simulink model "p1p2p3_Traking_Control"  (R2020b)
settings: Solver=FixedStepDiscrete  StartTime=0.0  StopTime=Inf  FixedStep=0.005  RelTol=1e-3  EnableMultiTasking=on
undefined symbols (not defined in the file or in its folder): DiscIntNeverNeededParam, Send_GUIdata, Writer
libraries: simulink x12, c280xlib x4, c2833xlib x4, dspsrcs4 x2, c2000lib x1
settings Model: ExtModeTrigDuration=8  Creator=Administrator  LastModifiedBy=Administrator
settings DataIOCC: ReturnWorkspaceOutputs=off
settings OptimizationCC: DefaultUnderspecifiedDataType=single  EnhancedBackFolding=on  PassReuseOutputArgsAs=Individual arguments  MaxStackSize=512  OptimizeBlockOrder=speed  DifferentSizesBufferReuse=on  OptimizationCustomize=off  EfficientTunableParamExpr=on
settings DebuggingCC: MultiTaskDSMMsg=none  ParameterTunabilityLossMsg=error  ArithmeticOperatorsInVariantConditions=warning
settings HardwareCC: ProdBitPerChar=16  ProdBitPerInt=16  ProdBitPerPointer=32  ProdBitPerSizeT=32  ProdBitPerPtrDiffT=32  ProdLargestAtomicInteger=Integer  ProdLargestAtomicFloat=None  ProdWordSize=16  ProdLongLongMode=on  ProdHWDeviceType=Texas Instruments->C2000
settings SFSimCC: MATLABDynamicMemAlloc=off  CustomCodeUndefinedFunction=UseInterfaceOnly
settings RTWCC: Description=Embedded Coder  SystemTargetFile=ert.tlc  HardwareBoard=TI Delfino F2833x  TemplateMakefile=ert_default_tmf  GenerateReport=on  Toolchain=Texas Instruments Code Composer Studio (C2000)  IncludeHyperlinkInReport=on  LaunchReport=on  GenerateTraceInfo=on  GenerateTraceReport=on  GenerateTraceReportSl=on  GenerateTraceReportSf=on  GenerateTraceReportEml=on
settings CodeAppCC: ForceParamTrailComments=on  IgnoreCustomStorageClasses=off  OperatorAnnotations=on  SimulinkDataObjDesc=on  SFDataObjDesc=on  InsertBlockDesc=on
settings ERTTargetCC: CodeReplacementLibrary=TI C28x

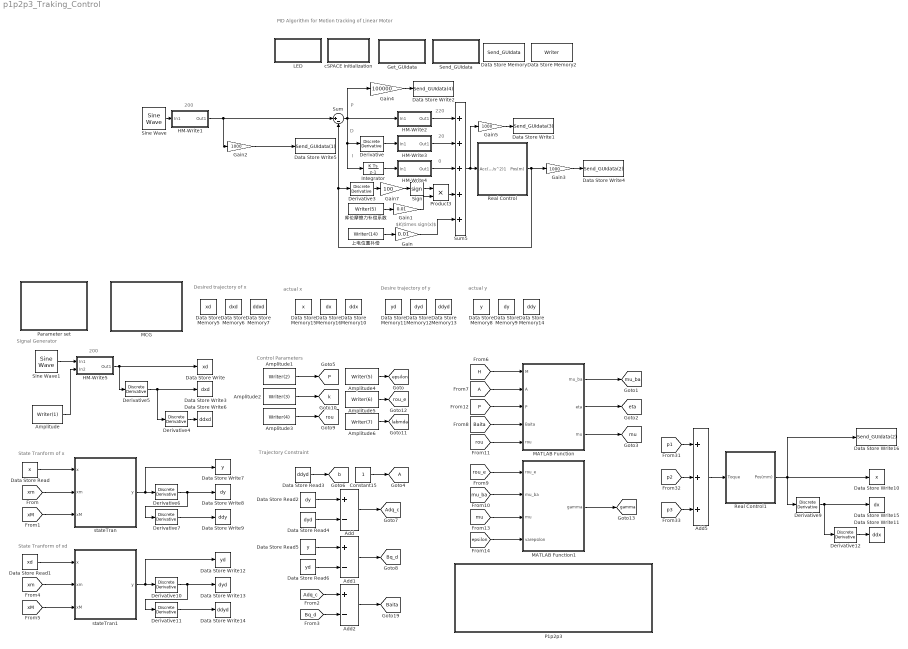
== system p1p2p3_Traking_Control ==
  note: 20
  note: 220
  note: PID Algorithm for Motion tracking of Linear Motor
  note: D
  note: I
  note: 200
  note: P
  note: $K\times sign(x)$
  note: 0
  note: Signal Generator
  note: State Tranform of x
  note: State Tranform of xd
  note: Desired trajectory of x
  note: actual y
  note: Control Parameters
  note: Desire trajectory of y
  note: Trajectory Constraint
  note: actual x
  note: 200
  Add : Sum  Inputs=+-
  Add1 : Sum  Inputs=+-
  Add2 : Sum  Inputs=+-
  Add5 : Sum  Inputs=+++
  Amplitude : DataStoreRead  DataStoreName=Writer  DataStoreElements=Writer(1)
  Amplitude1 : DataStoreRead  DataStoreName=Writer  DataStoreElements=Writer(2)
  Amplitude2 : DataStoreRead  DataStoreName=Writer  DataStoreElements=Writer(3)
  Amplitude3 : DataStoreRead  DataStoreName=Writer  DataStoreElements=Writer(4)
  Amplitude4 : DataStoreRead  DataStoreName=Writer  DataStoreElements=Writer(5)
  Amplitude5 : DataStoreRead  DataStoreName=Writer  DataStoreElements=Writer(6)
  Amplitude6 : DataStoreRead  DataStoreName=Writer  DataStoreElements=Writer(7)
  Constant15 : Constant
  Data Store Memory : DataStoreMemory  DataStoreName=Send_GUIdata  ReadBeforeWriteMsg=warning  WriteAfterWriteMsg=warning  WriteAfterReadMsg=warning  InitialValue=zeros(1,10)  ShowAdditionalParam=off
  Data Store Memory10 : DataStoreMemory  DataStoreName=ddx  ReadBeforeWriteMsg=warning  WriteAfterWriteMsg=warning  WriteAfterReadMsg=warning  ShowAdditionalParam=off
  Data Store Memory11 : DataStoreMemory  DataStoreName=yd  ReadBeforeWriteMsg=warning  WriteAfterWriteMsg=warning  WriteAfterReadMsg=warning  ShowAdditionalParam=off
  Data Store Memory12 : DataStoreMemory  DataStoreName=dyd  ReadBeforeWriteMsg=warning  WriteAfterWriteMsg=warning  WriteAfterReadMsg=warning  ShowAdditionalParam=off
  Data Store Memory13 : DataStoreMemory  DataStoreName=ddyd  ReadBeforeWriteMsg=warning  WriteAfterWriteMsg=warning  WriteAfterReadMsg=warning  ShowAdditionalParam=off
  Data Store Memory14 : DataStoreMemory  DataStoreName=ddy  ReadBeforeWriteMsg=warning  WriteAfterWriteMsg=warning  WriteAfterReadMsg=warning  ShowAdditionalParam=off
  Data Store Memory15 : DataStoreMemory  DataStoreName=x  ReadBeforeWriteMsg=warning  WriteAfterWriteMsg=warning  WriteAfterReadMsg=warning  ShowAdditionalParam=off
  Data Store Memory16 : DataStoreMemory  DataStoreName=dx  ReadBeforeWriteMsg=warning  WriteAfterWriteMsg=warning  WriteAfterReadMsg=warning  ShowAdditionalParam=off
  Data Store Memory2 : DataStoreMemory  DataStoreName=Writer  ReadBeforeWriteMsg=warning  WriteAfterWriteMsg=warning  WriteAfterReadMsg=warning  InitialValue=zeros(1,15)  ShowAdditionalParam=off  OutDataTypeStr=double
  Data Store Memory5 : DataStoreMemory  DataStoreName=xd  ReadBeforeWriteMsg=warning  WriteAfterWriteMsg=warning  WriteAfterReadMsg=warning  ShowAdditionalParam=off
  Data Store Memory6 : DataStoreMemory  DataStoreName=dxd  ReadBeforeWriteMsg=warning  WriteAfterWriteMsg=warning  WriteAfterReadMsg=warning  ShowAdditionalParam=off
  Data Store Memory7 : DataStoreMemory  DataStoreName=ddxd  ReadBeforeWriteMsg=warning  WriteAfterWriteMsg=warning  WriteAfterReadMsg=warning  ShowAdditionalParam=off
  Data Store Memory8 : DataStoreMemory  DataStoreName=y  ReadBeforeWriteMsg=warning  WriteAfterWriteMsg=warning  WriteAfterReadMsg=warning  ShowAdditionalParam=off
  Data Store Memory9 : DataStoreMemory  DataStoreName=dy  ReadBeforeWriteMsg=warning  WriteAfterWriteMsg=warning  WriteAfterReadMsg=warning  ShowAdditionalParam=off
  Data Store Read : DataStoreRead  DataStoreName=x
  Data Store Read1 : DataStoreRead  DataStoreName=xd
  Data Store Read2 : DataStoreRead  DataStoreName=dy
  Data Store Read3 : DataStoreRead  DataStoreName=ddyd
  Data Store Read4 : DataStoreRead  DataStoreName=dyd
  Data Store Read5 : DataStoreRead  DataStoreName=y
  Data Store Read6 : DataStoreRead  DataStoreName=yd
  Data Store Write : DataStoreWrite  DataStoreName=xd
  Data Store Write1 : DataStoreWrite  DataStoreName=Send_GUIdata  DataStoreElements=Send_GUIdata(3)
  Data Store Write10 : DataStoreWrite  DataStoreName=x
  Data Store Write11 : DataStoreWrite  DataStoreName=ddx
  Data Store Write12 : DataStoreWrite  DataStoreName=yd
  Data Store Write13 : DataStoreWrite  DataStoreName=dyd
  Data Store Write14 : DataStoreWrite  DataStoreName=ddyd
  Data Store Write15 : DataStoreWrite  DataStoreName=dx
  Data Store Write16 : DataStoreWrite  DataStoreName=Send_GUIdata  DataStoreElements=Send_GUIdata(2)
  Data Store Write2 : DataStoreWrite  DataStoreName=Send_GUIdata  DataStoreElements=Send_GUIdata(4)
  Data Store Write3 : DataStoreWrite  DataStoreName=dxd
  Data Store Write4 : DataStoreWrite  DataStoreName=Send_GUIdata  DataStoreElements=Send_GUIdata(2)
  Data Store Write5 : DataStoreWrite  DataStoreName=Send_GUIdata  DataStoreElements=Send_GUIdata(1)
  Data Store Write6 : DataStoreWrite  DataStoreName=ddxd
  Data Store Write7 : DataStoreWrite  DataStoreName=y
  Data Store Write8 : DataStoreWrite  DataStoreName=dy
  Data Store Write9 : DataStoreWrite  DataStoreName=ddy
  Derivative : simulink/Discrete/Discrete Derivative  gainval=1.0  ICPrevScaledInput=0.0  OutMin=[]  OutMax=[]  OutDataType=sfix(16)  OutScaling=2^-10  DoSatur=off
  Derivative{4..7,9..12} (8 alike) : simulink/Discrete/Discrete Derivative  gainval=1  ICPrevScaledInput=0.0  OutMin=[]  OutMax=[]  OutDataType=sfix(16)  OutScaling=2^-10  DoSatur=off
  Derivative3 : simulink/Discrete/Discrete Derivative  gainval=1.0  ICPrevScaledInput=0.0  OutMin=[]  OutMax=[]  OutDataType=sfix(16)  OutScaling=2^-10  DoSatur=off
  Gain : Gain  Gain=0.01
  Gain1 : Gain  Gain=0.01
  Gain2 : Gain  Gain=1000
  Gain3 : Gain  Gain=1000
  Gain4 : Gain  Gain=100000
  Gain5 : Gain  Gain=1000
  Gain7 : Gain  Gain=100
  Get_GUIdata : Subsystem
      mask Display: disp('从上位机获取\n控制数据')
  HM-Write1 : Subsystem
  HM-Write2 : Subsystem
  HM-Write3 : Subsystem
  HM-Write4 : Subsystem
  HM-Write5 : Subsystem
  Integrator : DiscreteIntegrator  SampleTime=-1  ICPrevOutput=DiscIntNeverNeededParam  ICPrevScaledInput=DiscIntNeverNeededParam
  LED : Subsystem  TreatAsAtomicUnit=on
      settings: RTWSystemCode=Nonreusable function
  MATLAB Function : MATLAB Function  TreatAsAtomicUnit=on
  MATLAB Function1 : MATLAB Function  TreatAsAtomicUnit=on
  "MCG " : Subsystem
  P1p2p3 : Subsystem  Priority=3
  Parameter set : Subsystem
  Product3 : Product
  Real Control : Subsystem
      mask Display:
      | port_label('input',1,'Acc(m/s^2)','texmode','on');
      | port_label('output',1,'Pos(m)','texmode','on');
  Real Control1 : Subsystem
  Send_GUIdata : Subsystem  mask{VChoice=4}
      mask prompts: VChoice "Select a variant choice"
      mask help: 选择发送几路通道的数据，“4”：表示发送数据到上位机的通道1~4；“10”：表示发送数据到上位机的通道1~10
      mask init:
      | simulationStatus =  get_param(bdroot,'SimulationStatus');
      | 
      | % The active variant can only be modified at edit-time or very early during
      | % the simulink compile stage. 
      | 
      |     choice = get_param(gcb,'VChoice');
      |     vssBlk = [gcb, '/VariantSubsystem'];
      |     oldVariant = get_param(gcb,'OverrideUsingVariant');
      | 
      |     if strcmp(choice,'4')
      | 
      |         set_param(vssBlk, 'OverrideUsingVariant', 'Variant1');
      |     else
      | 
      |         set_param(vssBlk, 'OverrideUsingVariant', 'Variant2');
      |     end
      mask TypeOptions VChoice: 4 | 10
      mask Display: disp('发送数据\n到上位机显示')
  Sign : Signum
  Sine Wave : dspsrcs4/Sine Wave  Amplitude=1  Frequency=1/4  Phase=0  SampleMode=Discrete  OutComplex=Real  CompMethod=Trigonometric fcn  TableSize=Speed  SampleTime=5/1000  SamplesPerFrame=1  ResetState=Restart at time zero  OutputFrames=off  dataType=double  wordLen=16  udDataType=sfix(16)  fracBitsMode=Best precision  numFracBits=15  OutDataTypeStr=double  LastOutDataTypeStr=double
  Sine Wave1 : dspsrcs4/Sine Wave  Amplitude=1  Frequency=1  Phase=0  SampleMode=Discrete  OutComplex=Real  CompMethod=Trigonometric fcn  TableSize=Speed  SampleTime=5/1000  SamplesPerFrame=1  ResetState=Restart at time zero  OutputFrames=off  dataType=double  wordLen=16  udDataType=sfix(16)  fracBitsMode=Best precision  numFracBits=15  OutDataTypeStr=double  LastOutDataTypeStr=double
  Sum : Sum  Inputs=|+-
  Sum5 : Sum  Inputs=5
  cSPACE Initialization : Subsystem  Priority=0
      mask Display: disp('Initialize \ncSPACE');
  stateTran : Subsystem
  stateTran1 : Subsystem
  上电位置补偿 : DataStoreRead  DataStoreName=Writer  DataStoreElements=Writer(14)
  库伦摩擦力补偿系数 : DataStoreRead  DataStoreName=Writer  DataStoreElements=Writer(5)
  tag scope: A=global, Adq_c=global, Baita=global, Bq_d=global, P=global, b=global, epsilon=global, eta=global, gamma=global, k=global, labmda=global, mu=global, mu_ba=global, rou=global, rou_e=global
  wires:
  Sum/1 -> HM-Write2/1(In1), Gain4/1, Integrator/1, Derivative/1
  Integrator/1 -> HM-Write4/1(In1)
  HM-Write2/1(Out1) -> Sum5/1
  HM-Write4/1(Out1) -> Sum5/3
  Sine Wave/1 -> HM-Write1/1(In1)
  Sum5/1 -> Gain5/1, Real Control/1(Acc(m/s^2)1)
  Derivative/1 -> HM-Write3/1(In1)
  HM-Write3/1(Out1) -> Sum5/2
  Gain7/1 -> Sign/1
  Real Control/1(Pos(m)) -> Gain3/1, Sum/2, Derivative3/1
  Gain1/1 -> Product3/2
  Sign/1 -> Product3/1
  库伦摩擦力补偿系数/1 -> Gain1/1
  Derivative3/1 -> Gain7/1
  Product3/1 -> Sum5/4
  上电位置补偿/1 -> Gain/1
  Gain/1 -> Sum5/5
  HM-Write1/1(Out1) -> Gain2/1, Sum/1
  Gain2/1 -> Data Store Write5/1
  Gain3/1 -> Data Store Write4/1
  Gain4/1 -> Data Store Write2/1
  Gain5/1 -> Data Store Write1/1
  Amplitude1/1 -> [P]
  Derivative12/1 -> Data Store Write11/1
  Data Store Read3/1 -> [b]
  Derivative9/1 -> Data Store Write15/1, Derivative12/1
  Derivative7/1 -> Data Store Write9/1
  Real Control1/1(Pos(mm)) -> Data Store Write16/1, Data Store Write10/1, Derivative9/1
  Derivative6/1 -> Derivative7/1, Data Store Write8/1
  Add5/1 -> Real Control1/1(Toque)
  [p3] -> Add5/3
  [rou] -> MATLAB Function/5(rou)
  [Bq_d] -> Add2/2
  [P] -> MATLAB Function/3(P)
  [xm] -> stateTran1/2(xm)
  [epsilon] -> MATLAB Function1/4(varepsilon)
  [p2] -> Add5/2
  MATLAB Function1/1(gamma) -> [gamma]
  [mu_ba] -> MATLAB Function1/2(mu_ba)
  Data Store Read1/1 -> stateTran1/1(x)
  Add/1 -> [Adq_c]
  HM-Write5/1(Out1) -> Data Store Write/1, Derivative5/1
  Sine Wave1/1 -> HM-Write5/1(In1)
  Amplitude3/1 -> [rou]
  Constant15/1 -> [A]
  Data Store Read2/1 -> Add/1
  Amplitude4/1 -> [epsilon]
  Derivative4/1 -> Data Store Write6/1
  MATLAB Function/3(mu) -> [mu]
  Amplitude2/1 -> [k]
  Derivative5/1 -> Data Store Write3/1, Derivative4/1
  [xM] -> stateTran1/3(xM)
  stateTran1/1(y) -> Data Store Write12/1, Derivative10/1
  [Baita] -> MATLAB Function/4(Baita)
  Data Store Read5/1 -> Add1/1
  [xm] -> stateTran/2(xm)
  Derivative10/1 -> Derivative11/1, Data Store Write13/1
  [H] -> MATLAB Function/1(M)
  Data Store Read4/1 -> Add/2
  MATLAB Function/1(mu_ba) -> [mu_ba]
  Derivative11/1 -> Data Store Write14/1
  stateTran/1(y) -> Data Store Write7/1, Derivative6/1
  Data Store Read/1 -> stateTran/1(x)
  Data Store Read6/1 -> Add1/2
  MATLAB Function/2(eta) -> [eta]
  [p1] -> Add5/1
  [Adq_c] -> Add2/1
  Add1/1 -> [Bq_d]
  [rou_e] -> MATLAB Function1/1(rou_e)
  Add2/1 -> [Baita]
  [mu] -> MATLAB Function1/3(mu)
  Amplitude/1 -> HM-Write5/2(In2)
  Amplitude5/1 -> [rou_e]
  [xM] -> stateTran/3(xM)
  Amplitude6/1 -> [labmda]
  [A] -> MATLAB Function/2(A)

== system p1p2p3_Traking_Control/Get_GUIdata ==
  Data Store Memory1 : DataStoreMemory  DataStoreName=Get_GUIData  ReadBeforeWriteMsg=warning  WriteAfterWriteMsg=warning  WriteAfterReadMsg=warning  InitialValue=zeros(1,15)  ShowAdditionalParam=off
  Data Store Read5 : DataStoreRead  DataStoreName=Get_GUIData
  Data Store Write : DataStoreWrite  DataStoreName=Writer
  SCIA RCV Interrupt : c2000lib/Scheduling/C28x Hardware Interrupt  irqnumbers=9  pienumbers=1  irqpriorities=1  irqpreempts=0  showinput=off  dspchiptype=C280X
      settings: SourceProductBaseCode=TIC2000
  Subsystem : Subsystem
  wires:
  SCIA RCV Interrupt/1 -> Subsystem/Trigger
  Data Store Read5/1 -> Data Store Write/1

== system p1p2p3_Traking_Control/HM-Write1 ==
  In1 : Inport
  Product5 : Product
  gain : Gain  Gain=0.001  OutDataTypeStr=double
  幅值 : DataStoreRead  DataStoreName=Writer  DataStoreElements=Writer(1)
  Out1 : Outport  VectorParamsAs1DForOutWhenUnconnected=off
  wires:
  In1/1 -> Product5/1
  Product5/1 -> Out1/1
  幅值/1 -> gain/1
  gain/1 -> Product5/2

== system p1p2p3_Traking_Control/HM-Write2 ==
  In1 : Inport
  Gain5 : Gain  Gain=0.1  OutDataTypeStr=double
  Kp : DataStoreRead  DataStoreName=Writer  DataStoreElements=Writer(2)
  Product1 : Product
  Out1 : Outport  VectorParamsAs1DForOutWhenUnconnected=off
  wires:
  In1/1 -> Product1/1
  Product1/1 -> Out1/1
  Gain5/1 -> Product1/2
  Kp/1 -> Gain5/1

== system p1p2p3_Traking_Control/HM-Write3 ==
  In1 : Inport
  Gain3 : Gain  Gain=0.1  OutDataTypeStr=double
  KD : DataStoreRead  DataStoreName=Writer  DataStoreElements=Writer(3)
  Product6 : Product
  Out1 : Outport  VectorParamsAs1DForOutWhenUnconnected=off
  wires:
  Gain3/1 -> Product6/2
  KD/1 -> Gain3/1
  Product6/1 -> Out1/1
  In1/1 -> Product6/1

== system p1p2p3_Traking_Control/HM-Write4 ==
  In1 : Inport
  Gain2 : Gain  Gain=0.1  OutDataTypeStr=double
  KD : DataStoreRead  DataStoreName=Writer  DataStoreElements=Writer(4)
  Product2 : Product
  Out1 : Outport  VectorParamsAs1DForOutWhenUnconnected=off
  wires:
  Product2/1 -> Out1/1
  KD/1 -> Gain2/1
  Gain2/1 -> Product2/2
  In1/1 -> Product2/1

== system p1p2p3_Traking_Control/HM-Write5 ==
  In1 : Inport
  In2 : Inport  Port=2
  Product5 : Product
  gain : Gain  Gain=0.01  OutDataTypeStr=double
  Out1 : Outport  VectorParamsAs1DForOutWhenUnconnected=off
  wires:
  gain/1 -> Product5/2
  Product5/1 -> Out1/1
  In1/1 -> Product5/1
  In2/1 -> gain/1

== system p1p2p3_Traking_Control/LED ==
  note: get
  CTC : simulink/Logic and Bit Operations/Compare To Constant  relop=<=  const=200  OutDataTypeStr=boolean
  Counter : simulink/Sources/Counter Limited  uplimit=400  tsamp=-1
  GPIO14 : c2833xlib/Digital Output  GPIO_Number=GPIO8~GPIO15  GPIO_Bit0=off  GPIO_BIT0_Toggle=off  GPIO_Bit1=off  GPIO_BIT1_Toggle=off  GPIO_Bit2=off  GPIO_BIT2_Toggle=off  GPIO_Bit3=off  GPIO_BIT3_Toggle=off  GPIO_Bit4=off  GPIO_BIT4_Toggle=off  GPIO_Bit5=off  GPIO_BIT5_Toggle=off  GPIO_Bit6=on  GPIO_BIT6_Toggle=off  GPIO_Bit7=off  GPIO_BIT7_Toggle=off
      settings: SourceProductBaseCode=TIC2000
  wires:
  Counter/1 -> CTC/1
  CTC/1 -> GPIO14/1

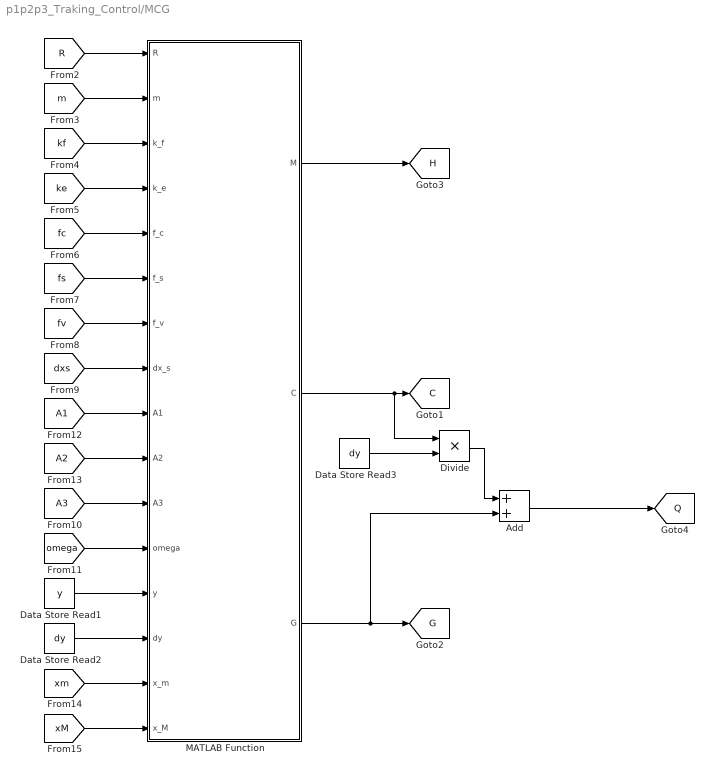
== system p1p2p3_Traking_Control/MCG  ==
  Add : Sum
  Data Store Read1 : DataStoreRead  DataStoreName=y
  Data Store Read2 : DataStoreRead  DataStoreName=dy
  Data Store Read3 : DataStoreRead  DataStoreName=dy
  Divide : Product  Inputs=**
  MATLAB Function : MATLAB Function  TreatAsAtomicUnit=on
  tag scope: C=global, G=global, H=global, Q=global
  wires:
  [A2] -> MATLAB Function/10(A2)
  [ke] -> MATLAB Function/4(k_e)
  [dxs] -> MATLAB Function/8(dx_s)
  MATLAB Function/2(C) -> Divide/1, [C]
  MATLAB Function/3(G) -> [G], Add/2
  [omega] -> MATLAB Function/12(omega)
  [fc] -> MATLAB Function/5(f_c)
  [fs] -> MATLAB Function/6(f_s)
  Data Store Read2/1 -> MATLAB Function/14(dy)
  [kf] -> MATLAB Function/3(k_f)
  [m] -> MATLAB Function/2(m)
  MATLAB Function/1(M) -> [H]
  [R] -> MATLAB Function/1(R)
  [A3] -> MATLAB Function/11(A3)
  [xm] -> MATLAB Function/15(x_m)
  [A1] -> MATLAB Function/9(A1)
  [xM] -> MATLAB Function/16(x_M)
  Data Store Read1/1 -> MATLAB Function/13(y)
  [fv] -> MATLAB Function/7(f_v)
  Add/1 -> [Q]
  Divide/1 -> Add/1
  Data Store Read3/1 -> Divide/2

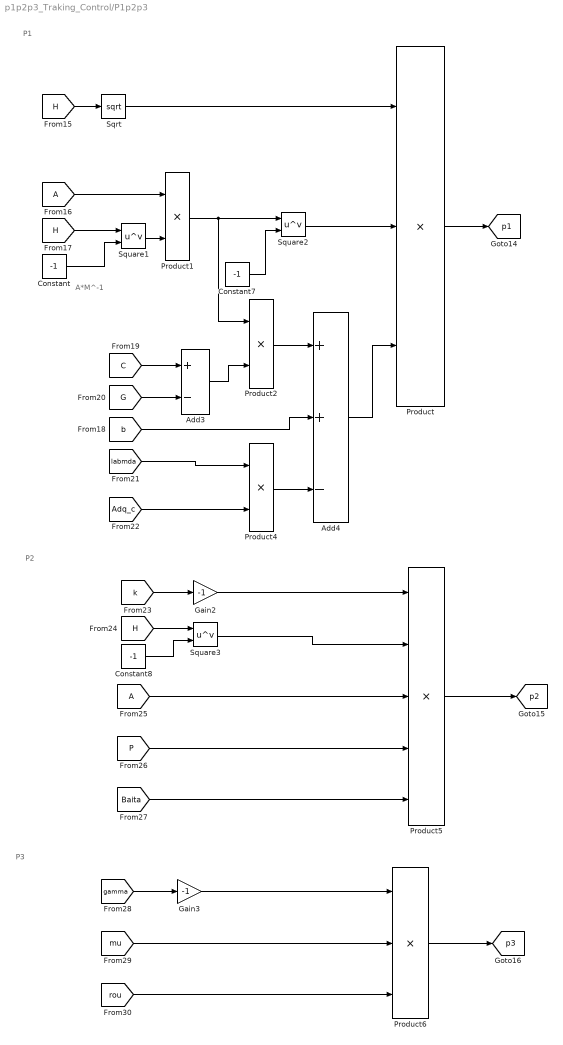
== system p1p2p3_Traking_Control/P1p2p3 ==
  note: P3
  note: P1
  note: A*M^-1
  note: P2
  Add3 : Sum  Inputs=+-
  Add4 : Sum  Inputs=++-
  Constant : Constant  Value=-1
  Constant7 : Constant  Value=-1
  Constant8 : Constant  Value=-1
  Gain2 : Gain  Gain=-1
  Gain3 : Gain  Gain=-1
  Product : Product  Inputs=3
  Product1 : Product
  Product2 : Product
  Product4 : Product
  Product5 : Product  Inputs=5
  Product6 : Product  Inputs=3
  Sqrt : Sqrt  SaturateOnIntegerOverflow=on
  Square1 : Math  Operator=pow  SaturateOnIntegerOverflow=on
  Square2 : Math  Operator=pow  SaturateOnIntegerOverflow=on
  Square3 : Math  Operator=pow  SaturateOnIntegerOverflow=on
  tag scope: p1=global, p2=global, p3=global
  wires:
  Constant/1 -> Square1/2
  Product2/1 -> Add4/1
  Square2/1 -> Product/2
  [A] -> Product1/1
  Product5/1 -> [p2]
  Product/1 -> [p1]
  [Adq_c] -> Product4/2
  [H] -> Square3/1
  Product1/1 -> Product2/1, Square2/1
  [H] -> Square1/1
  [mu] -> Product6/2
  [G] -> Add3/2
  Square3/1 -> Product5/2
  Square1/1 -> Product1/2
  [k] -> Gain2/1
  [A] -> Product5/3
  Gain2/1 -> Product5/1
  Constant7/1 -> Square2/2
  [H] -> Sqrt/1
  Sqrt/1 -> Product/1
  [C] -> Add3/1
  [gamma] -> Gain3/1
  Add4/1 -> Product/3
  [b] -> Add4/2
  Product6/1 -> [p3]
  Product4/1 -> Add4/3
  Gain3/1 -> Product6/1
  Add3/1 -> Product2/2
  [rou] -> Product6/3
  [Baita] -> Product5/5
  [P] -> Product5/4
  [labmda] -> Product4/1
  Constant8/1 -> Square3/2

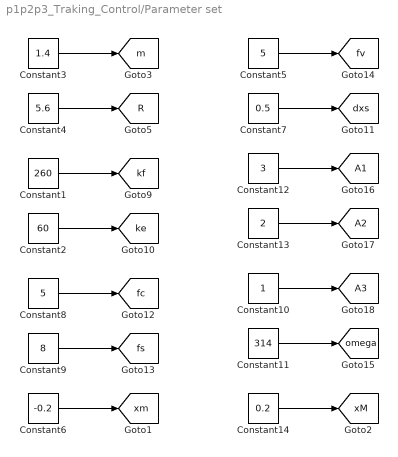
== system p1p2p3_Traking_Control/Parameter set ==
  Constant1 : Constant  Value=260
  Constant10 : Constant
  Constant11 : Constant  Value=314
  Constant12 : Constant  Value=3
  Constant13 : Constant  Value=2
  Constant14 : Constant  Value=0.2
  Constant2 : Constant  Value=60
  Constant3 : Constant  Value=1.4
  Constant4 : Constant  Value=5.6
  Constant5 : Constant  Value=5
  Constant6 : Constant  Value=-0.2
  Constant7 : Constant  Value=0.5
  Constant8 : Constant  Value=5
  Constant9 : Constant  Value=8
  tag scope: A1=global, A2=global, A3=global, R=global, dxs=global, fc=global, fs=global, fv=global, ke=global, kf=global, m=global, omega=global, xM=global, xm=global
  wires:
  Constant4/1 -> [R]
  Constant3/1 -> [m]
  Constant1/1 -> [kf]
  Constant2/1 -> [ke]
  Constant7/1 -> [dxs]
  Constant5/1 -> [fv]
  Constant8/1 -> [fc]
  Constant9/1 -> [fs]
  Constant13/1 -> [A2]
  Constant10/1 -> [A3]
  Constant11/1 -> [omega]
  Constant12/1 -> [A1]
  Constant6/1 -> [xm]
  Constant14/1 -> [xM]

== system p1p2p3_Traking_Control/Real Control ==
  Acc(m/s^2)1 : Inport
  Get Cart's Position : Subsystem  TreatAsAtomicUnit=on
      mask help:
      | 小车的位置分辨率:1um/脉冲
      | 位置单位：m
      settings: RTWSystemCode=Nonreusable function
      mask Display: disp('Get Position');
  "Set Cart's Acc " : Subsystem
      mask help: 将加速度通过数字电压转换成最终的模拟电压驱使小车移动
      mask Display:
      | disp('          SetAcc');
      | port_label('input', 1, 'Acc(m/s^2)');
  Pos(m) : Outport  VectorParamsAs1DForOutWhenUnconnected=off
  wires:
  Get Cart's Position/1(Pos(m)) -> Pos(m)/1
  Acc(m/s^2)1/1 -> "Set Cart's Acc "/1(In1)

== system p1p2p3_Traking_Control/Real Control1 ==
  Toque : Inport
  Gain10 : Gain  Gain=1000
  GetCart'sPosition : Subsystem  TreatAsAtomicUnit=on
      mask help:
      | 小车的位置分辨率:1um/脉冲
      | 位置单位：m
      settings: RTWSystemCode=Nonreusable function
      mask Display: disp('Get Position');
  "Set Cart's Toq " : Subsystem
      mask help: 将加速度通过数字电压转换成最终的模拟电压驱使小车移动
      mask Display:
      | disp('          SetToq');
      | port_label('input', 1, 'Toque');
  Pos(mm) : Outport  VectorParamsAs1DForOutWhenUnconnected=off
  wires:
  GetCart'sPosition/1(Pos(m)) -> Gain10/1
  Toque/1 -> "Set Cart's Toq "/1(In1)
  Gain10/1 -> Pos(mm)/1

== system p1p2p3_Traking_Control/Send_GUIdata ==
  Data Store Read20 : DataStoreRead  DataStoreName=Send_GUIdata
  VariantSubsystem : Subsystem  Variant=on  VariantControlMode=label  LabelModeActiveChoice=Variant1
  wires:
  Data Store Read20/1 -> VariantSubsystem/1(In1)

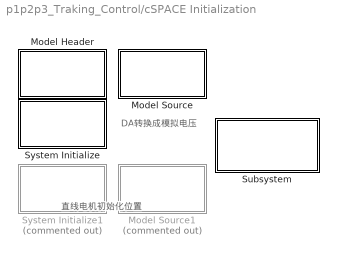
== system p1p2p3_Traking_Control/cSPACE Initialization ==
  note: DA转换成模拟电压
  note: 直线电机初始化位置
  Model Header : Subsystem  mask(Model Header){ShowInLibBrowser=0}
      mask prompts: ShowInLibBrowser "Mask Parameter 1:"
      mask help: Add code to the model .h file
      settings: CopyFcn=cccopyfcn(gcb)  OpenFcn=ccopenfcn('Model Header')
      mask Help: eval('feval(''rtwprivate'',''rtwhelpview'',''rtw_model_header_block'')');
      mask Display: disp('Model\nHeader');
  Model Source : Subsystem  mask(Model Source){ShowInLibBrowser=0}
      mask prompts: ShowInLibBrowser "Mask Parameter 1:"
      mask help: Add code to the model .c file
      settings: CopyFcn=cccopyfcn(gcb)  OpenFcn=ccopenfcn('Model Source')
      mask Help: helpview([docroot '/toolbox/rtw/helptargets.map'], 'rtw_model_source_block');
      mask Display: disp('Model\nSource');
  Model Source1 : Subsystem  Commented=on  mask(Model Source){ShowInLibBrowser=0}
      mask prompts: ShowInLibBrowser "Mask Parameter 1:"
      mask help: Add code to the model .c file
      settings: CopyFcn=cccopyfcn(gcb)  OpenFcn=ccopenfcn('Model Source')
      mask Help: eval('feval(''rtwprivate'',''rtwhelpview'',''rtw_model_source_block'')');
      mask Display: disp('Model\nSource');
  Subsystem : Subsystem  TreatAsAtomicUnit=on
      settings: RTWSystemCode=Nonreusable function
      mask Display: disp('Elmo驱动器IO复位')
  System Initialize : Subsystem  mask(System Initialize){ShowInLibBrowser=0}
      mask prompts: ShowInLibBrowser "Mask Parameter 1:"
      mask help: Add code to a systems Initialize function
      settings: CopyFcn=cccopyfcn(gcb)  OpenFcn=ccopenfcn('System Initialize Function')
      mask Help: helpview([docroot '/toolbox/rtw/helptargets.map'], 'rtw_sys_initialize_block');
      mask Display: disp('System\nInitialize');
  System Initialize1 : Subsystem  Commented=on  mask(System Initialize){ShowInLibBrowser=0}
      mask prompts: ShowInLibBrowser "Mask Parameter 1:"
      mask help: Add code to a systems Initialize function
      settings: CopyFcn=cccopyfcn(gcb)  OpenFcn=ccopenfcn('System Initialize Function')
      mask Help: eval('feval(''rtwprivate'',''rtwhelpview'',''rtw_sys_initialize_block'')');
      mask Display: disp('System\nInitialize');

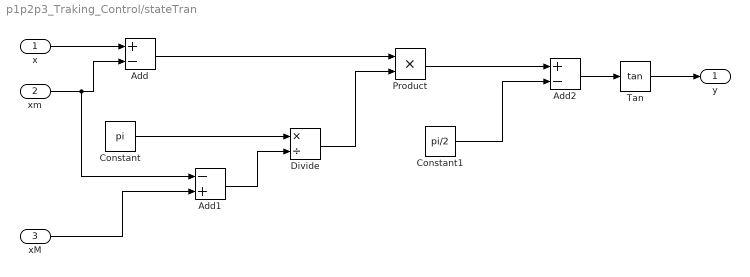
== system p1p2p3_Traking_Control/stateTran ==
  x : Inport
  xm : Inport  Port=2
  xM : Inport  Port=3
  Add : Sum  Inputs=+-
  Add1 : Sum  Inputs=-+
  Add2 : Sum  Inputs=+-
  Constant : Constant  Value=pi
  Constant1 : Constant  Value=pi/2
  Divide : Product  Inputs=*/
  Product : Product
  Tan : Trigonometry  Operator=tan
  y : Outport
  wires:
  Constant/1 -> Divide/1
  xm/1 -> Add1/1, Add/2
  Add1/1 -> Divide/2
  xM/1 -> Add1/2
  Constant1/1 -> Add2/2
  Divide/1 -> Product/2
  Product/1 -> Add2/1
  Add/1 -> Product/1
  Add2/1 -> Tan/1
  x/1 -> Add/1
  Tan/1 -> y/1

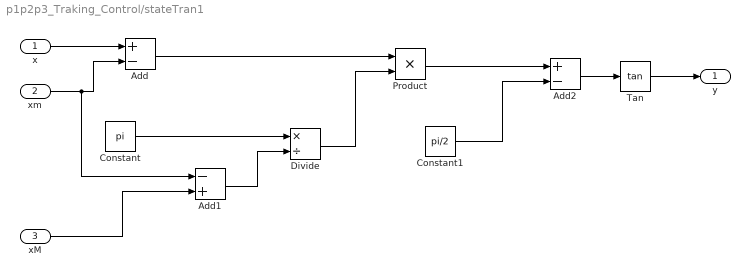
== system p1p2p3_Traking_Control/stateTran1 ==
  x : Inport
  xm : Inport  Port=2
  xM : Inport  Port=3
  Add : Sum  Inputs=+-
  Add1 : Sum  Inputs=-+
  Add2 : Sum  Inputs=+-
  Constant : Constant  Value=pi
  Constant1 : Constant  Value=pi/2
  Divide : Product  Inputs=*/
  Product : Product
  Tan : Trigonometry  Operator=tan
  y : Outport
  wires:
  Constant/1 -> Divide/1
  xm/1 -> Add1/1, Add/2
  Add1/1 -> Divide/2
  xM/1 -> Add1/2
  Constant1/1 -> Add2/2
  Divide/1 -> Product/2
  Product/1 -> Add2/1
  Add/1 -> Product/1
  Add2/1 -> Tan/1
  x/1 -> Add/1
  Tan/1 -> y/1

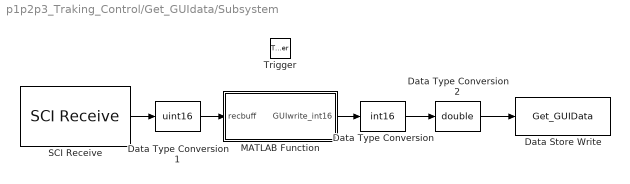
== system p1p2p3_Traking_Control/Get_GUIdata/Subsystem ==
  Trigger : TriggerPort  TriggerType=function-call  VariantControl=Variant  PortDimensions=1
  Data Store Write : DataStoreWrite  DataStoreName=Get_GUIData
  Data Type Conversion : DataTypeConversion  OutDataTypeStr=int16
  Data Type Conversion1 : DataTypeConversion  OutDataTypeStr=uint16
  Data Type Conversion2 : DataTypeConversion  OutDataTypeStr=double
  MATLAB Function : MATLAB Function  TreatAsAtomicUnit=on
  SCI Receive : c280xlib/SCI Receive  sciModule=A  dataHead=''  dataTail=''  dataType=uint8  dataDim=32  initValue=0  errOption=Output the last received value  errValue=0  sampleTime=-1  outputStatus=off  postInterrupt=on  numFifo=16
      settings: SourceProductBaseCode=TIC2000
  wires:
  SCI Receive/1 -> Data Type Conversion1/1
  MATLAB Function/1(GUIwrite_int16) -> Data Type Conversion/1
  Data Type Conversion1/1 -> MATLAB Function/1(recbuff)
  Data Type Conversion/1 -> Data Type Conversion2/1
  Data Type Conversion2/1 -> Data Store Write/1

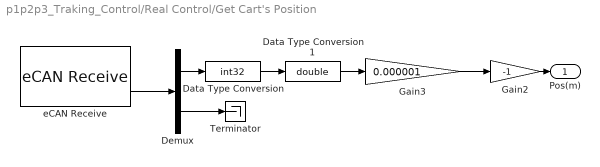
== system p1p2p3_Traking_Control/Real Control/Get Cart's Position ==
  Data Type Conversion : DataTypeConversion  OutDataTypeStr=int32
  Data Type Conversion1 : DataTypeConversion  OutDataTypeStr=double
  Demux : Demux  Outputs=2
  Gain2 : Gain  Gain=-1
  Gain3 : Gain  Gain=0.000001
  Terminator : Terminator
  eCAN Receive : c280xlib/eCAN Receive  chipFamily=C280x  useModule=eCAN_A  mailboxNo=0  messageID=1  messageType=Standard (11-bit identifier)  sampleTime=-1  dataType=uint32  initValue=0  outputMessageLength=off  outputMessageTimeStamp=off  postInterrupt=off  interruptLine=0
      settings: SourceProductBaseCode=TIC2000
  Pos(m) : Outport  VectorParamsAs1DForOutWhenUnconnected=off
  wires:
  eCAN Receive/2 -> Demux/1
  Demux/1 -> Data Type Conversion/1
  Data Type Conversion/1 -> Data Type Conversion1/1
  Demux/2 -> Terminator/1
  Gain3/1 -> Gain2/1
  Gain2/1 -> Pos(m)/1
  Data Type Conversion1/1 -> Gain3/1

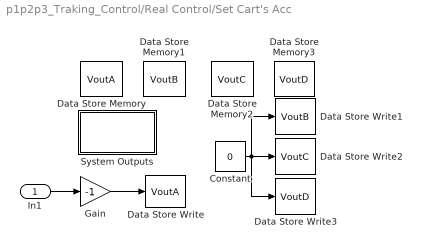
== system p1p2p3_Traking_Control/Real Control/Set Cart's Acc  ==
  In1 : Inport
  Constant : Constant  Value=0
  Data Store Memory : DataStoreMemory  DataStoreName=VoutA  ReadBeforeWriteMsg=warning  WriteAfterWriteMsg=warning  WriteAfterReadMsg=warning  ShowAdditionalParam=off
  Data Store Memory1 : DataStoreMemory  DataStoreName=VoutB  ReadBeforeWriteMsg=warning  WriteAfterWriteMsg=warning  WriteAfterReadMsg=warning  ShowAdditionalParam=off
  Data Store Memory2 : DataStoreMemory  DataStoreName=VoutC  ReadBeforeWriteMsg=warning  WriteAfterWriteMsg=warning  WriteAfterReadMsg=warning  ShowAdditionalParam=off
  Data Store Memory3 : DataStoreMemory  DataStoreName=VoutD  ReadBeforeWriteMsg=warning  WriteAfterWriteMsg=warning  WriteAfterReadMsg=warning  ShowAdditionalParam=off
  Data Store Write : DataStoreWrite  DataStoreName=VoutA
  Data Store Write1 : DataStoreWrite  DataStoreName=VoutB
  Data Store Write2 : DataStoreWrite  DataStoreName=VoutC
  Data Store Write3 : DataStoreWrite  DataStoreName=VoutD
  Gain : Gain  Gain=-1
  System Outputs : Subsystem  mask(System Outputs){ShowInLibBrowser=0}
      mask prompts: ShowInLibBrowser "Mask Parameter 1:"
      mask help: Add code to a systems Outputs function
      settings: CopyFcn=cccopyfcn(gcb)  OpenFcn=ccopenfcn('System Outputs Function')
      mask Help: helpview([docroot '/toolbox/rtw/helptargets.map'], 'rtw_sys_outputs_block');
      mask Display: disp('System\nOutputs');
  wires:
  Constant/1 -> Data Store Write3/1, Data Store Write2/1, Data Store Write1/1
  In1/1 -> Gain/1
  Gain/1 -> Data Store Write/1

== system p1p2p3_Traking_Control/Real Control1/GetCart'sPosition ==
  Data Store Read : DataStoreRead  DataStoreName=Motor_Position
  Gain1 : Gain  Gain=-0.000001
  Pos(m) : Outport  VectorParamsAs1DForOutWhenUnconnected=off
  wires:
  Gain1/1 -> Pos(m)/1
  Data Store Read/1 -> Gain1/1

== system p1p2p3_Traking_Control/Real Control1/Set Cart's Toq  ==
  In1 : Inport
  Data Store Write : DataStoreWrite  DataStoreName=Motor_Tor
  wires:
  In1/1 -> Data Store Write/1

== system p1p2p3_Traking_Control/Send_GUIdata/VariantSubsystem ==
  note: 1) Add Subsystem or Model blocks as valid variant choices.
      | 2) You cannot connect blocks at this level. At simulation, connectivity is automatically
      | determined, based on the active variant and port name matching.
  In1 : Inport
  Send10 : Subsystem  TreatAsAtomicUnit=on  VariantControl=Variant2
      settings: RTWSystemCode=Nonreusable function
  Srnd4 : Subsystem  TreatAsAtomicUnit=on  VariantControl=Variant1
      settings: RTWSystemCode=Nonreusable function

== system p1p2p3_Traking_Control/cSPACE Initialization/Model Header ==

== system p1p2p3_Traking_Control/cSPACE Initialization/Model Source ==

== system p1p2p3_Traking_Control/cSPACE Initialization/Model Source1 ==

== system p1p2p3_Traking_Control/cSPACE Initialization/Subsystem ==
  note: Elmo IO复位
  note: 28035 复位
  Constant : Constant
  Digital Output34 : c2833xlib/Digital Output  GPIO_Number=GPIO32~GPIO39  GPIO_Bit0=off  GPIO_BIT0_Toggle=off  GPIO_Bit1=off  GPIO_BIT1_Toggle=off  GPIO_Bit2=on  GPIO_BIT2_Toggle=off  GPIO_Bit3=off  GPIO_BIT3_Toggle=off  GPIO_Bit4=off  GPIO_BIT4_Toggle=off  GPIO_Bit5=off  GPIO_BIT5_Toggle=off  GPIO_Bit6=off  GPIO_BIT6_Toggle=off  GPIO_Bit7=off  GPIO_BIT7_Toggle=off
      settings: SourceProductBaseCode=TIC2000
  Digital Output35 : c2833xlib/Digital Output  GPIO_Number=GPIO32~GPIO39  GPIO_Bit0=off  GPIO_BIT0_Toggle=off  GPIO_Bit1=off  GPIO_BIT1_Toggle=off  GPIO_Bit2=off  GPIO_BIT2_Toggle=off  GPIO_Bit3=on  GPIO_BIT3_Toggle=off  GPIO_Bit4=off  GPIO_BIT4_Toggle=off  GPIO_Bit5=off  GPIO_BIT5_Toggle=off  GPIO_Bit6=off  GPIO_BIT6_Toggle=off  GPIO_Bit7=off  GPIO_BIT7_Toggle=off
      settings: SourceProductBaseCode=TIC2000
  Digital Output36 : c2833xlib/Digital Output  GPIO_Number=GPIO32~GPIO39  GPIO_Bit0=off  GPIO_BIT0_Toggle=off  GPIO_Bit1=off  GPIO_BIT1_Toggle=off  GPIO_Bit2=off  GPIO_BIT2_Toggle=off  GPIO_Bit3=off  GPIO_BIT3_Toggle=off  GPIO_Bit4=on  GPIO_BIT4_Toggle=off  GPIO_Bit5=off  GPIO_BIT5_Toggle=off  GPIO_Bit6=off  GPIO_BIT6_Toggle=off  GPIO_Bit7=off  GPIO_BIT7_Toggle=off
      settings: SourceProductBaseCode=TIC2000
  Step : Step  Time=0.5  SampleTime=0.005
  wires:
  Constant/1 -> Digital Output35/1, Digital Output36/1
  Step/1 -> Digital Output34/1

== system p1p2p3_Traking_Control/cSPACE Initialization/System Initialize ==

== system p1p2p3_Traking_Control/cSPACE Initialization/System Initialize1 ==

== system p1p2p3_Traking_Control/Real Control/Set Cart's Acc /System Outputs ==

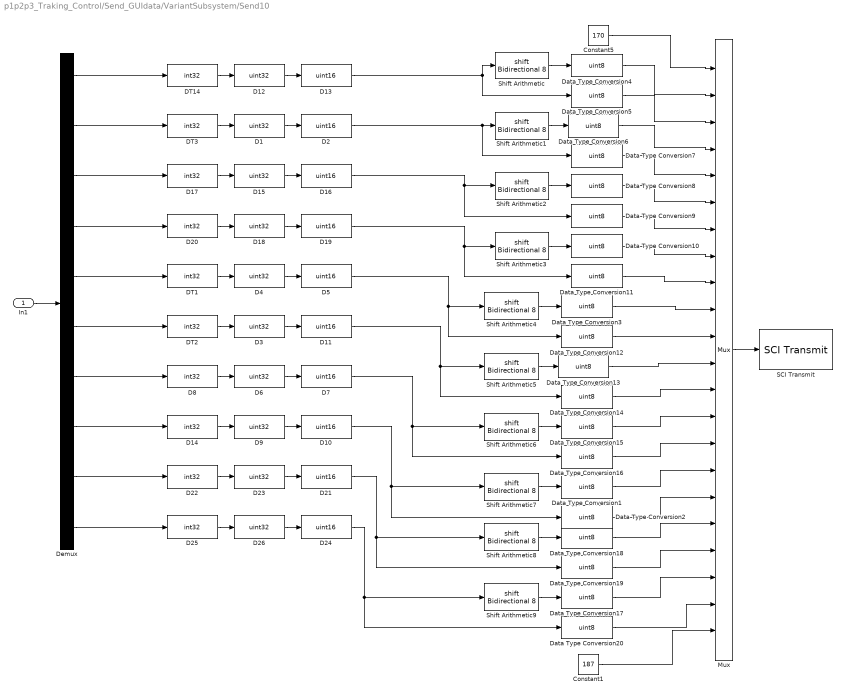
== system p1p2p3_Traking_Control/Send_GUIdata/VariantSubsystem/Send10 ==
  In1 : Inport
  Constant1 : Constant  Value=187  OutDataTypeStr=uint8
  Constant5 : Constant  Value=170  OutDataTypeStr=uint8
  D{1,3..4,6,9,12,15,18,23,26} (10 alike) : DataTypeConversion  OutDataTypeStr=uint32
  D{2,5,7,10..11,13,16,19,21,24} (10 alike) : DataTypeConversion  OutDataTypeStr=uint16
  D{8,14,17,20,22,25} (6 alike) : DataTypeConversion  OutDataTypeStr=int32
  DT{1..3,14} (4 alike) : DataTypeConversion  OutDataTypeStr=int32
  Data Type Conversion{1..20} (20 alike) : DataTypeConversion  OutDataTypeStr=uint8
  Demux : Demux  Outputs=10
  Mux : Mux  Inputs=22
  SCI Transmit : c280xlib/SCI Transmit  sciModule=A  dataHead=''  dataTail=''  postInterrupt=on  numFifo=16
  Shift Arithmetic{,1..9} (10 alike) : ArithShift  BitShiftNumber=8
  wires:
  Demux/10 -> D25/1
  Demux/9 -> D22/1
  In1/1 -> Demux/1
  Demux/1 -> DT14/1
  Data Type Conversion11/1 -> Mux/9
  D12/1 -> D13/1
  Data Type Conversion9/1 -> Mux/7
  DT3/1 -> D1/1
  DT14/1 -> D12/1
  Shift Arithmetic2/1 -> Data Type Conversion8/1
  Data Type Conversion7/1 -> Mux/5
  Shift Arithmetic/1 -> Data Type Conversion4/1
  D15/1 -> D16/1
  D20/1 -> D18/1
  Data Type Conversion8/1 -> Mux/6
  D17/1 -> D15/1
  D18/1 -> D19/1
  D2/1 -> Shift Arithmetic1/1, Data Type Conversion7/1
  Data Type Conversion4/1 -> Mux/2
  Shift Arithmetic3/1 -> Data Type Conversion10/1
  Constant5/1 -> Mux/1
  Data Type Conversion6/1 -> Mux/4
  D19/1 -> Data Type Conversion11/1, Shift Arithmetic3/1
  Shift Arithmetic1/1 -> Data Type Conversion6/1
  Data Type Conversion5/1 -> Mux/3
  Mux/1 -> SCI Transmit/1
  Demux/4 -> D20/1
  D1/1 -> D2/1
  Demux/2 -> DT3/1
  Data Type Conversion10/1 -> Mux/8
  D16/1 -> Data Type Conversion9/1, Shift Arithmetic2/1
  Demux/3 -> D17/1
  D13/1 -> Data Type Conversion5/1, Shift Arithmetic/1
  D5/1 -> Data Type Conversion12/1, Shift Arithmetic4/1
  Data Type Conversion1/1 -> Mux/16
  Data Type Conversion12/1 -> Mux/11
  Shift Arithmetic5/1 -> Data Type Conversion13/1
  D10/1 -> Shift Arithmetic7/1, Data Type Conversion2/1
  Data Type Conversion13/1 -> Mux/12
  Shift Arithmetic7/1 -> Data Type Conversion1/1
  Data Type Conversion3/1 -> Mux/10
  D11/1 -> Data Type Conversion14/1, Shift Arithmetic5/1
  Data Type Conversion15/1 -> Mux/14
  Shift Arithmetic4/1 -> Data Type Conversion3/1
  Data Type Conversion14/1 -> Mux/13
  Shift Arithmetic6/1 -> Data Type Conversion15/1
  Data Type Conversion16/1 -> Mux/15
  Data Type Conversion2/1 -> Mux/17
  Demux/6 -> DT2/1
  D3/1 -> D11/1
  Demux/8 -> D14/1
  D9/1 -> D10/1
  D8/1 -> D6/1
  D14/1 -> D9/1
  D6/1 -> D7/1
  DT1/1 -> D4/1
  DT2/1 -> D3/1
  D4/1 -> D5/1
  Demux/7 -> D8/1
  D7/1 -> Shift Arithmetic6/1, Data Type Conversion16/1
  D22/1 -> D23/1
  D23/1 -> D21/1
  D26/1 -> D24/1
  D25/1 -> D26/1
  Demux/5 -> DT1/1
  Data Type Conversion20/1 -> Mux/21
  Data Type Conversion19/1 -> Mux/19
  Shift Arithmetic8/1 -> Data Type Conversion18/1
  Data Type Conversion18/1 -> Mux/18
  Shift Arithmetic9/1 -> Data Type Conversion17/1
  D24/1 -> Shift Arithmetic9/1, Data Type Conversion20/1
  Data Type Conversion17/1 -> Mux/20
  D21/1 -> Shift Arithmetic8/1, Data Type Conversion19/1
  Constant1/1 -> Mux/22

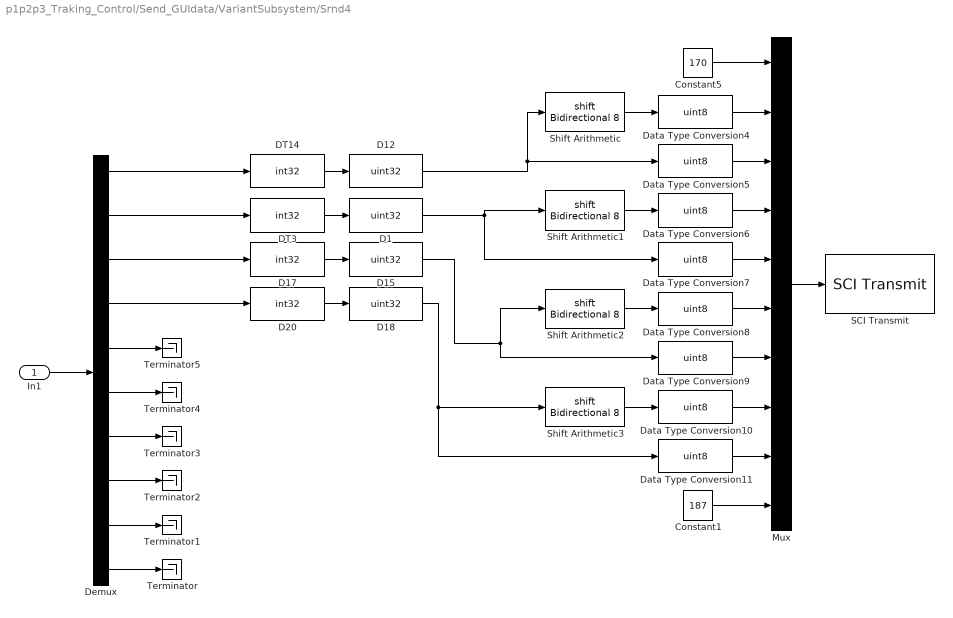
== system p1p2p3_Traking_Control/Send_GUIdata/VariantSubsystem/Srnd4 ==
  In1 : Inport
  Constant1 : Constant  Value=187  OutDataTypeStr=uint8
  Constant5 : Constant  Value=170  OutDataTypeStr=uint8
  D{1,12,15,18} (4 alike) : DataTypeConversion  OutDataTypeStr=uint32
  D17 : DataTypeConversion  OutDataTypeStr=int32
  D20 : DataTypeConversion  OutDataTypeStr=int32
  DT14 : DataTypeConversion  OutDataTypeStr=int32
  DT3 : DataTypeConversion  OutDataTypeStr=int32
  Data Type Conversion{4..11} (8 alike) : DataTypeConversion  OutDataTypeStr=uint8
  Demux : Demux  Outputs=10
  Mux : Mux  Inputs=10
  SCI Transmit : c280xlib/SCI Transmit  sciModule=A  dataHead=''  dataTail=''  postInterrupt=on  numFifo=16
  Shift Arithmetic{,1..3} (4 alike) : ArithShift  BitShiftNumber=8
  Terminator{,1..5} (6 alike) : Terminator
  wires:
  In1/1 -> Demux/1
  Demux/3 -> D17/1
  Demux/1 -> DT14/1
  Demux/2 -> DT3/1
  Demux/4 -> D20/1
  Demux/10 -> Terminator/1
  Demux/9 -> Terminator1/1
  Demux/8 -> Terminator2/1
  Demux/7 -> Terminator3/1
  Demux/6 -> Terminator4/1
  Demux/5 -> Terminator5/1
  DT14/1 -> D12/1
  DT3/1 -> D1/1
  D17/1 -> D15/1
  D20/1 -> D18/1
  Data Type Conversion11/1 -> Mux/9
  Data Type Conversion9/1 -> Mux/7
  Shift Arithmetic2/1 -> Data Type Conversion8/1
  Data Type Conversion7/1 -> Mux/5
  D18/1 -> Data Type Conversion11/1, Shift Arithmetic3/1
  D1/1 -> Data Type Conversion7/1, Shift Arithmetic1/1
  Shift Arithmetic/1 -> Data Type Conversion4/1
  Data Type Conversion8/1 -> Mux/6
  Constant1/1 -> Mux/10
  Data Type Conversion4/1 -> Mux/2
  Shift Arithmetic3/1 -> Data Type Conversion10/1
  Data Type Conversion6/1 -> Mux/4
  Constant5/1 -> Mux/1
  Mux/1 -> SCI Transmit/1
  D15/1 -> Data Type Conversion9/1, Shift Arithmetic2/1
  D12/1 -> Shift Arithmetic/1, Data Type Conversion5/1
  Data Type Conversion5/1 -> Mux/3
  Data Type Conversion10/1 -> Mux/8
  Shift Arithmetic1/1 -> Data Type Conversion6/1

== matlab function p1p2p3_Traking_Control/Get_GUIdata/Subsystem/MATLAB Function ==
  data: recbuff input; GUIwrite_int16 output
function GUIwrite_int16 = fcn(recbuff)
    GUIwrite_int16=[0 0 0 0 0 0 0 0 0 0 0 0 0 0 0];
    GUIwrite_int16(1)= recbuff(2)*256+recbuff(3);
    GUIwrite_int16(2)= recbuff(4)*256+recbuff(5);
    GUIwrite_int16(3)= recbuff(6)*256+recbuff(7);
    GUIwrite_int16(4)= recbuff(8)*256+recbuff(9);
    GUIwrite_int16(5)= recbuff(10)*256+recbuff(11);
    GUIwrite_int16(6)= recbuff(12)*256+recbuff(13);
    GUIwrite_int16(7)= recbuff(14)*256+recbuff(15);
    GUIwrite_int16(8)= recbuff(16)*256+recbuff(17);
    GUIwrite_int16(9)= recbuff(18)*256+recbuff(19);
    GUIwrite_int16(10)= recbuff(20)*256+recbuff(21);
    GUIwrite_int16(11)= recbuff(22)*256+recbuff(23);
    GUIwrite_int16(12)= recbuff(24)*256+recbuff(25);
    GUIwrite_int16(13)= recbuff(26)*256+recbuff(27);
    GUIwrite_int16(14)= recbuff(28)*256+recbuff(29);
    GUIwrite_int16(15)= recbuff(30)*256+recbuff(31);
end

== matlab function p1p2p3_Traking_Control/MCG /MATLAB Function ==
  data: R input; M output; m input; k_f input; k_e input; f_c input; f_s input; f_v input; dx_s input; A1 input; A2 input; A3 input; omega input; y input; dy input; x_m input; x_M input; C output; G output
function [M,C,G] = fcn(R,m,k_f,k_e,f_c,f_s,f_v,dx_s,A1,A2,A3,omega,y,dy,x_m,x_M)

%  R=5.6;          %系统阻抗
% m_ba=1.4;    %名义质量
% k_f=260;       %力矩常数
% k_e=60;        %反电动势
% f_c=5;           %库伦摩擦系数
% f_s=8;           %静摩擦力系数
% f_v=5;           %粘滞摩擦力系数
% dx_s=0.5;      %润滑条件
% A1=3;           %摩擦力第一项
% A2=2;           %摩擦力第二项
% A3=1;           %摩擦力第三项
% omega=314;  %摩擦力频率

      M_be_ba=R*m/k_f;

%       F_f=(f_c+(f_s-f_c)*(exp(1)^(-((x_M-x_m)*(sout(ka,2))/(pi*(1+(sout(ka,1))^2))/dx_s)^2)))*sign((x_M-x_m)*sout(ka,2)/(pi*(1+(sout(ka,1))^2)));
      F_f=(f_c+(f_s-f_c)*(exp(1)^(-((x_M-x_m)*(dy)/(pi*(1+(y)^2))/dx_s)^2)))*sign((x_M-x_m)*dy/(pi*(1+(y)^2)));
      F_r=A1*sin(omega*((x_M-x_m)*atan(y)/pi+(x_M+x_m)/2))+A2*sin(3*omega*((x_M-x_m)*atan(y)/pi+(x_M+x_m)/2))+A3*sin(5*omega*((x_M-x_m)*atan(y)/pi+(x_M+x_m)/2));
      F_d=0;
      F_l=0;
      F_e=F_f+F_r+F_d+F_l; 
      M=M_be_ba*(x_M-x_m)*(1+(y)^2)/(pi*(1+(y)^2)^2);
      C=(k_e+f_v)*(x_M-x_m)/(pi*(1+(y)^2));
      G=F_e-2*M_be_ba*(x_M-x_m)*((y)^2)*dy^2/(pi*(1+(y)^2)^2);
end

== matlab function p1p2p3_Traking_Control/MATLAB Function ==
  data: M input; mu_ba output; A input; P input; Baita input; rou input; eta output; mu output
function [mu_ba,eta,mu] = fcn(M,A,P,Baita,rou)
      mu_ba=M^(-1)*A'*P;
      eta=mu_ba*Baita;
      mu=eta*rou;

== matlab function p1p2p3_Traking_Control/MATLAB Function1 ==
  data: rou_e input; gamma output; mu_ba input; mu input; varepsilon input
function gamma= fcn(rou_e,mu_ba,mu,varepsilon)

if norm(mu)>varepsilon
        gamma=(1+rou_e)^(-1)/(norm(mu_ba)*norm(mu));
    else
        gamma=(1+rou_e)^(-1)/(norm(mu_ba)*norm(mu_ba)*varepsilon);
end
end
